simulink model "controller_plant_model"  (R2018b)
settings: Solver=VariableStepAuto  StartTime=0.0  StopTime=10.0  RelTol=1e-3
settings Model: Creator=Cole  LastModifiedBy=Cole

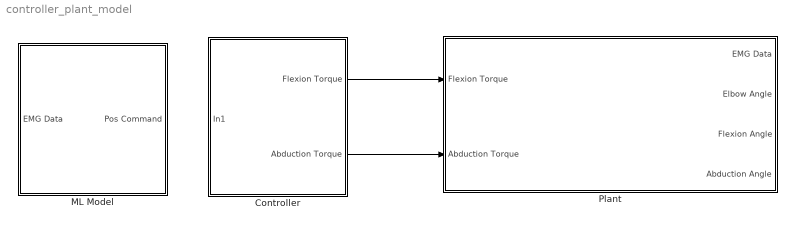
== system controller_plant_model ==
  Controller : Subsystem
  ML Model : Subsystem
  Plant : Subsystem
  wires:
  Controller/2(Abduction Torque) -> Plant/2(Abduction Torque)
  Controller/1(Flexion Torque) -> Plant/1(Flexion Torque)

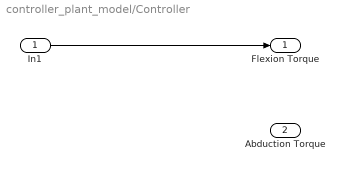
== system controller_plant_model/Controller ==
  In1 : Inport
  Flexion Torque : Outport
  Abduction Torque : Outport  Port=2
  wires:
  In1/1 -> Flexion Torque/1

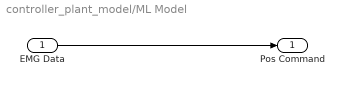
== system controller_plant_model/ML Model ==
  EMG Data : Inport
  Pos Command : Outport
  wires:
  EMG Data/1 -> Pos Command/1

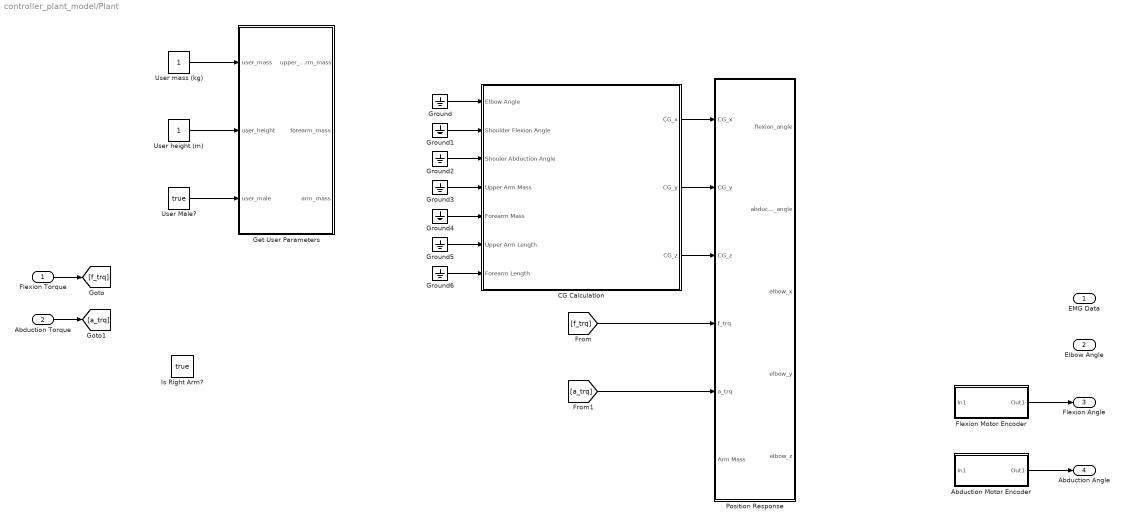
== system controller_plant_model/Plant ==
  Flexion Torque : Inport
  Abduction Torque : Inport  Port=2
  Abduction Motor Encoder : Subsystem
  CG Calculation : Subsystem
  Flexion Motor Encoder : Subsystem
  Get User Parameters : MATLAB Function  TreatAsAtomicUnit=on
  Ground{,1..6} (7 alike) : Ground
  Is Right Arm? : Constant  Value=true
  Position Response : Subsystem
  User Male? : Constant  Value=true
  User height (m) : Constant
  User mass (kg) : Constant
  EMG Data : Outport
  Elbow Angle : Outport  Port=2
  Flexion Angle : Outport  Port=3
  Abduction Angle : Outport  Port=4
  wires:
  User Male?/1 -> Get User Parameters/3(user_male)
  CG Calculation/2(CG_y) -> Position Response/2(CG_y)
  User mass (kg)/1 -> Get User Parameters/1(user_mass)
  User height (m)/1 -> Get User Parameters/2(user_height)
  CG Calculation/1(CG_x) -> Position Response/1(CG_x)
  Ground/1 -> CG Calculation/1(Elbow Angle)
  Ground1/1 -> CG Calculation/2(Shoulder Flexion Angle)
  Ground2/1 -> CG Calculation/3(Shouler Abduction Angle)
  Ground3/1 -> CG Calculation/4(Upper Arm Mass)
  Ground4/1 -> CG Calculation/5(Forearm Mass)
  Ground5/1 -> CG Calculation/6(Upper Arm Length)
  Ground6/1 -> CG Calculation/7(Forearm Length)
  Flexion Torque/1 -> [f_trq]
  Abduction Torque/1 -> [a_trq]
  [f_trq] -> Position Response/4(f_trq)
  [a_trq] -> Position Response/5(a_trq)
  CG Calculation/3(CG_z) -> Position Response/3(CG_z)
  Abduction Motor Encoder/1(Out1) -> Abduction Angle/1
  Flexion Motor Encoder/1(Out1) -> Flexion Angle/1

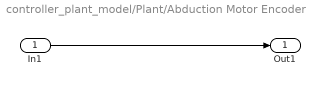
== system controller_plant_model/Plant/Abduction Motor Encoder ==
  In1 : Inport
  Out1 : Outport
  wires:
  In1/1 -> Out1/1

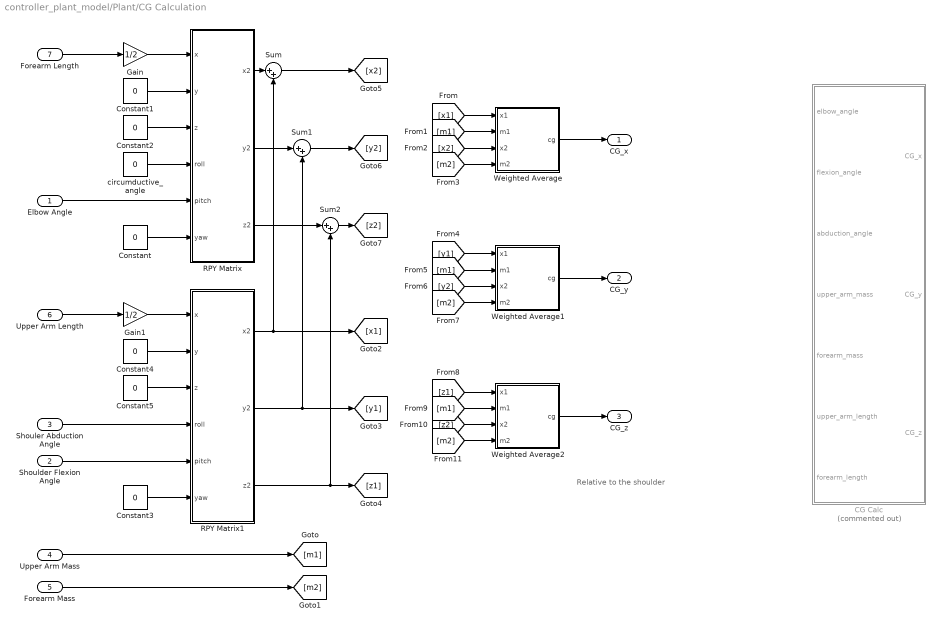
== system controller_plant_model/Plant/CG Calculation ==
  note: Relative to the shoulder
  Elbow Angle : Inport
  Shoulder Flexion Angle : Inport  Port=2
  Shouler Abduction Angle : Inport  Port=3
  Upper Arm Mass : Inport  Port=4
  Forearm Mass : Inport  Port=5
  Upper Arm Length : Inport  Port=6
  Forearm Length : Inport  Port=7
  CG Calc : MATLAB Function  Commented=on  TreatAsAtomicUnit=on
  Constant{,1..5} (6 alike) : Constant  Value=0
  Gain : Gain  Gain=1/2
  Gain1 : Gain  Gain=1/2
  RPY Matrix : MATLAB Function  TreatAsAtomicUnit=on
  RPY Matrix1 : MATLAB Function  TreatAsAtomicUnit=on
  Sum : Sum  Inputs=|++
  Sum1 : Sum  Inputs=|++
  Sum2 : Sum  Inputs=|++
  Weighted Average : MATLAB Function  TreatAsAtomicUnit=on
  Weighted Average1 : MATLAB Function  TreatAsAtomicUnit=on
  Weighted Average2 : MATLAB Function  TreatAsAtomicUnit=on
  circumductive_angle : Constant  Value=0
  CG_x : Outport
  CG_y : Outport  Port=2
  CG_z : Outport  Port=3
  wires:
  Elbow Angle/1 -> RPY Matrix/5(pitch)
  Forearm Length/1 -> Gain/1
  circumductive_angle/1 -> RPY Matrix/4(roll)
  Constant/1 -> RPY Matrix/6(yaw)
  Gain/1 -> RPY Matrix/1(x)
  Constant1/1 -> RPY Matrix/2(y)
  Constant2/1 -> RPY Matrix/3(z)
  Shouler Abduction Angle/1 -> RPY Matrix1/4(roll)
  Shoulder Flexion Angle/1 -> RPY Matrix1/5(pitch)
  Constant3/1 -> RPY Matrix1/6(yaw)
  Upper Arm Length/1 -> Gain1/1
  Gain1/1 -> RPY Matrix1/1(x)
  Constant4/1 -> RPY Matrix1/2(y)
  Constant5/1 -> RPY Matrix1/3(z)
  Weighted Average/1(cg) -> CG_x/1
  Weighted Average1/1(cg) -> CG_y/1
  Weighted Average2/1(cg) -> CG_z/1
  Upper Arm Mass/1 -> [m1]
  Forearm Mass/1 -> [m2]
  RPY Matrix1/1(x2) -> Sum/2, [x1]
  RPY Matrix1/2(y2) -> [y1], Sum1/2
  RPY Matrix1/3(z2) -> Sum2/2, [z1]
  RPY Matrix/1(x2) -> Sum/1
  RPY Matrix/2(y2) -> Sum1/1
  RPY Matrix/3(z2) -> Sum2/1
  [x1] -> Weighted Average/1(x1)
  [m1] -> Weighted Average/2(m1)
  [x2] -> Weighted Average/3(x2)
  [m2] -> Weighted Average/4(m2)
  [y1] -> Weighted Average1/1(x1)
  [m1] -> Weighted Average1/2(m1)
  [y2] -> Weighted Average1/3(x2)
  [m2] -> Weighted Average1/4(m2)
  [z1] -> Weighted Average2/1(x1)
  [m1] -> Weighted Average2/2(m1)
  [z2] -> Weighted Average2/3(x2)
  [m2] -> Weighted Average2/4(m2)
  Sum/1 -> [x2]
  Sum1/1 -> [y2]
  Sum2/1 -> [z2]

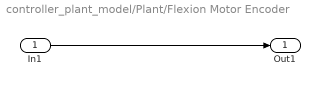
== system controller_plant_model/Plant/Flexion Motor Encoder ==
  In1 : Inport
  Out1 : Outport
  wires:
  In1/1 -> Out1/1

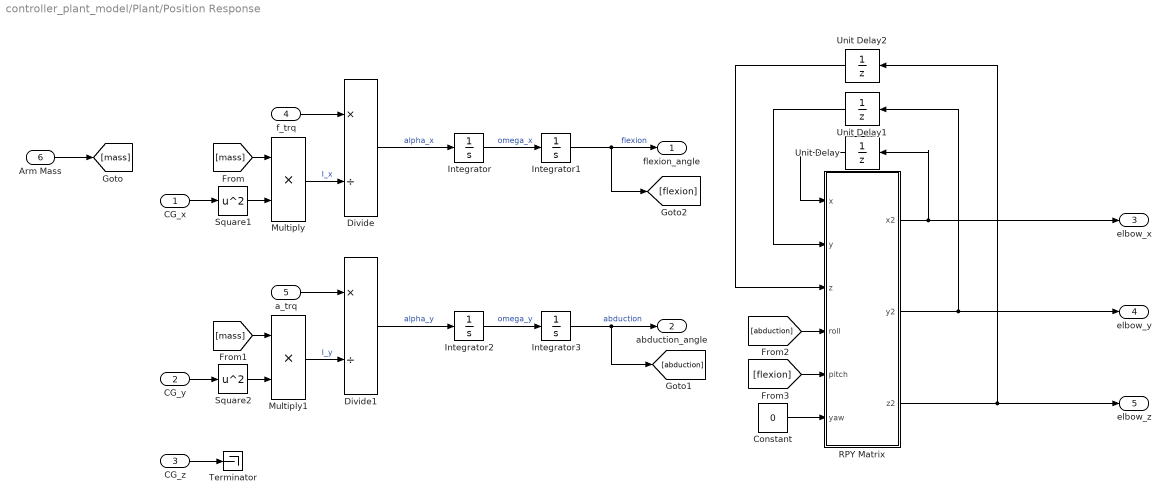
== system controller_plant_model/Plant/Position Response ==
  CG_x : Inport
  CG_y : Inport  Port=2
  CG_z : Inport  Port=3
  f_trq : Inport  Port=4
  a_trq : Inport  Port=5
  Arm Mass : Inport  Port=6
  Constant : Constant  Value=0
  Divide : Product  Inputs=*/
  Divide1 : Product  Inputs=*/
  Integrator{,1..3} (4 alike) : Integrator
  Multiply : Product
  Multiply1 : Product
  RPY Matrix : MATLAB Function  TreatAsAtomicUnit=on
  Square1 : Math  Operator=square  SaturateOnIntegerOverflow=on
  Square2 : Math  Operator=square  SaturateOnIntegerOverflow=on
  Terminator : Terminator
  Unit Delay : UnitDelay  SampleTime=-1
  Unit Delay1 : UnitDelay  SampleTime=-1
  Unit Delay2 : UnitDelay  SampleTime=-1
  flexion_angle : Outport
  abduction_angle : Outport  Port=2
  elbow_x : Outport  Port=3
  elbow_y : Outport  Port=4
  elbow_z : Outport  Port=5
  wires:
  CG_x/1 -> Square1/1
  Square1/1 -> Multiply/2
  Multiply/1 -> Divide/2  "I_x"
  f_trq/1 -> Divide/1
  Divide/1 -> Integrator/1  "alpha_x"
  Integrator/1 -> Integrator1/1  "omega_x"
  Integrator1/1 -> [flexion], flexion_angle/1  "flexion"
  Arm Mass/1 -> [mass]
  [mass] -> Multiply/1
  a_trq/1 -> Divide1/1
  Multiply1/1 -> Divide1/2  "I_y"
  Integrator3/1 -> [abduction], abduction_angle/1  "abduction"
  Divide1/1 -> Integrator2/1  "alpha_y"
  Integrator2/1 -> Integrator3/1  "omega_y"
  [mass] -> Multiply1/1
  Square2/1 -> Multiply1/2
  CG_y/1 -> Square2/1
  CG_z/1 -> Terminator/1
  [abduction] -> RPY Matrix/4(roll)
  [flexion] -> RPY Matrix/5(pitch)
  Constant/1 -> RPY Matrix/6(yaw)
  RPY Matrix/1(x2) -> Unit Delay/1, elbow_x/1
  RPY Matrix/2(y2) -> Unit Delay1/1, elbow_y/1
  RPY Matrix/3(z2) -> elbow_z/1, Unit Delay2/1
  Unit Delay/1 -> RPY Matrix/1(x)
  Unit Delay1/1 -> RPY Matrix/2(y)
  Unit Delay2/1 -> RPY Matrix/3(z)

== matlab function controller_plant_model/Plant/CG Calculation/CG Calc ==
  data: CG_x output; CG_y output; CG_z output; elbow_angle input; flexion_angle input; abduction_angle input; upper_arm_mass input; forearm_mass input; upper_arm_length input; forearm_length input
function [CG_x, CG_y, CG_z]= fcn(elbow_angle, flexion_angle, abduction_angle, upper_arm_mass, forearm_mass, upper_arm_length, forearm_length)

circumductive_angle = 0;

R_x =   [1 0 0;
        0 cos(abduction_angle) -sin(abduction_angle);
        0 sin(abduction_angle) cos(abduction_angle)];

R_y =   [cos(flexion_angle) 0 sin(flexion_angle);
        0 1 0;
        -sin(flexion_angle) 0 cos(flexion_angle)];

R_z = eye(3);

R_tot = R_x*R_y*R_z;

init_elbow_cg = [upper_arm_length/2 0 0];

final_elbow_cg = init_elbow_cg*R_tot;

R_x2 =  [1 0 0;
        0 cos(circumductive_angle) -sin(circumductive_angle);
        0 sin(circumductive_angle) cos(circumductive_angle)];

R_y2 =  [cos(elbow_angle) 0 sin(elbow_angle);
        0 1 0;
        -sin(elbow_angle) 0 cos(elbow_angle)];

R_z2 = eye(3);

R_tot2 = R_x2*R_y2*R_z2;

init_hand_cg = [forearm_length/2 0 0];
final_hand_cg = init_hand_cg*R_tot2;

CG_x = (final_elbow_cg(1)*upper_arm_mass + final_hand_cg(1)*forearm_mass)...
    / (upper_arm_mass+forearm_mass);
CG_y = (final_elbow_cg(2)*upper_arm_mass + final_hand_cg(2)*forearm_mass)...
    / (upper_arm_mass+forearm_mass);
CG_z = (final_elbow_cg(3)*upper_arm_mass + final_hand_cg(3)*forearm_mass)...
    / (upper_arm_mass+forearm_mass);
end

%{
elbow_x = upper_arm_length*sin(flexion_angle);
elbow_y = -upper_arm_length*sin(abduction_angle);
elbow_z = -upper_arm_length*sqrt(cos(flexion_angle)^2 + cos(abduction_angle)^2)/sqrt(2);

hand_x = forearm_length*cos(;
hand_y = 0;
hand_z = 0;
%}

== matlab function controller_plant_model/Plant/Get User Parameters ==
  data: user_mass input; user_height input; upper_arm_mass output; user_male input; forearm_mass output; arm_mass output
function [upper_arm_mass,forearm_mass,arm_mass] = fcn(user_mass, user_height, user_male)

if user_male
    upper_arm_mass = 0.0325*user_mass;
    forearm_mass = 0.0252*user_mass;
    arm_mass = upper_arm_mass + forearm_mass;
else
    upper_arm_mass = 0.029*user_mass;
    forearm_mass = 0.0207*user_mass;
    arm_mass = upper_arm_mass + forearm_mass;
end

== matlab function controller_plant_model/Plant/CG Calculation/RPY Matrix ==
  data: x input; y input; z input; roll input; x2 output; pitch input; yaw input; y2 output; z2 output
function [x2,y2,z2] = fcn(x,y,z,roll,pitch,yaw)

R_x =   [1 0 0;
        0 cos(roll) -sin(roll);
        0 sin(roll) cos(roll)];

R_y =   [cos(pitch) 0 sin(pitch);
        0 1 0;
        -sin(pitch) 0 cos(pitch)];

R_z =   [cos(yaw) -sin(yaw) 0
        sin(yaw) cos(yaw) 0
        0 0 1];

R_tot = R_x*R_y*R_z;

final_pos = [x y z]*R_tot;

x2 = final_pos(1);
y2 = final_pos(2);
z2 = final_pos(3);

== matlab function controller_plant_model/Plant/CG Calculation/RPY Matrix1 ==
  data: x input; y input; z input; roll input; x2 output; pitch input; yaw input; y2 output; z2 output
function [x2,y2,z2] = fcn(x,y,z,roll,pitch,yaw)

R_x =   [1 0 0;
        0 cos(roll) -sin(roll);
        0 sin(roll) cos(roll)];

R_y =   [cos(pitch) 0 sin(pitch);
        0 1 0;
        -sin(pitch) 0 cos(pitch)];

R_z =   [cos(yaw) -sin(yaw) 0
        sin(yaw) cos(yaw) 0
        0 0 1];

R_tot = R_x*R_y*R_z;

final_pos = [x y z]*R_tot;

x2 = final_pos(1);
y2 = final_pos(2);
z2 = final_pos(3);

== matlab function controller_plant_model/Plant/CG Calculation/Weighted Average ==
  data: x1 input; cg output; m1 input; x2 input; m2 input
function cg = fcn(x1,m1,x2,m2)

cg = (x1*m1 + x2*m2) / (m1+m2);

== matlab function controller_plant_model/Plant/CG Calculation/Weighted Average1 ==
  data: x1 input; cg output; m1 input; x2 input; m2 input
function cg = fcn(x1,m1,x2,m2)

cg = (x1*m1 + x2*m2) / (m1+m2);

== matlab function controller_plant_model/Plant/CG Calculation/Weighted Average2 ==
  data: x1 input; cg output; m1 input; x2 input; m2 input
function cg = fcn(x1,m1,x2,m2)

cg = (x1*m1 + x2*m2) / (m1+m2);

== matlab function controller_plant_model/Plant/Position Response/RPY Matrix ==
  data: x input; y input; z input; roll input; x2 output; pitch input; yaw input; y2 output; z2 output
function [x2,y2,z2] = fcn(x,y,z,roll,pitch,yaw)

R_x =   [1 0 0;
        0 cos(roll) -sin(roll);
        0 sin(roll) cos(roll)];

R_y =   [cos(pitch) 0 sin(pitch);
        0 1 0;
        -sin(pitch) 0 cos(pitch)];

R_z =   [cos(yaw) -sin(yaw) 0
        sin(yaw) cos(yaw) 0
        0 0 1];

R_tot = R_x*R_y*R_z;

final_pos = [x y z]*R_tot;

x2 = final_pos(1);
y2 = final_pos(2);
z2 = final_pos(3);
